simulink model "prob09"  (R2020b)
settings: Solver=VariableStepAuto  StartTime=0.0  StopTime=10.0  RelTol=1e-3
libraries: simulink x6, powerlib x5, sdolib x1
settings Model: Creator=stkaravind  LastModifiedBy=stkaravind

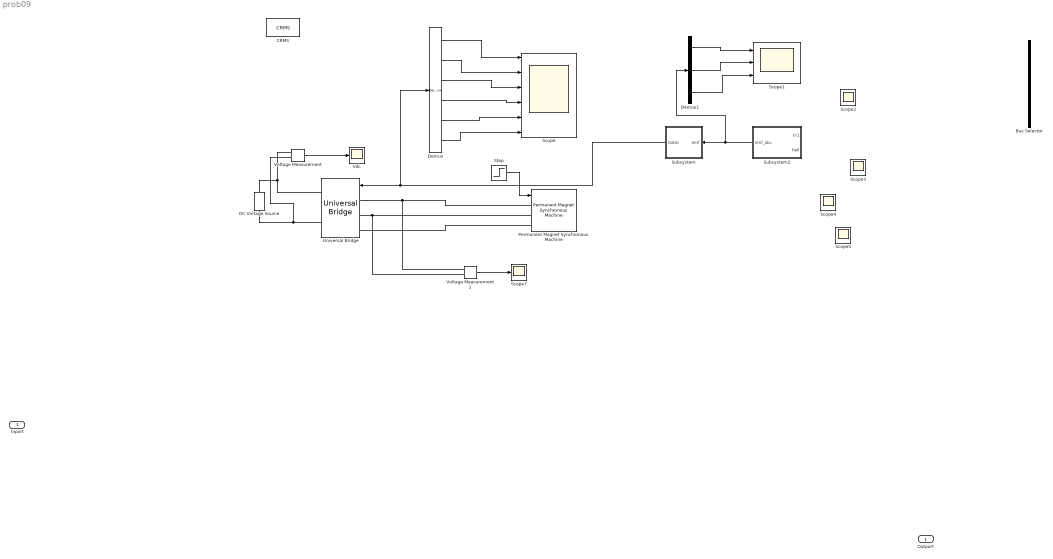
== system prob09 ==
  Inport : Inport
  Bus Selector : BusSelector  OutputSignals=signal1,signal2
  CRMS : sdolib/RMS Blocks/CRMS
      settings: SourceProductBaseCode=SO
  DC Voltage Source : powerlib/Electrical Sources/DC Voltage Source  Amplitude=300  Measurements=None
  Demux : Demux  Outputs=6
  Demux1 : Demux  Outputs=3
  Permanent Magnet Synchronous Machine : powerlib/Machines/Permanent Magnet Synchronous Machine  NbPhases=3  FluxDistribution=Trapezoidal  RotorType=Round  MechanicalLoad=Torque Tm  PresetModel=No  ShowDetailedParameters=on  MeasurementBus=off  Resistance=0.0485  Inductance=8.5e-3  dqInductances=[8.5e-3,8.5e-3]  La=0.000395  MachineConstant=Flux linkage established by magnets (V.s)  Flux=0.1194  VoltageCst=100.0283  TorqueCst=0.9552  Flat=120  Mechanical=[0.0027 0.0004924 4 0]  PolePairs=4  InitialConditions=[0,0, 0,0]  InitialConditions5ph=[0 0 0 0 0 0]  RefAngle=90 degrees behind phase A axis (modified Park)  IterativeDiscreteModel=Trapezoidal non iterative  TsBlock=-1  TsPowergui=0
  Scope : Scope  NumInputPorts=6
  Scope1 : Scope  NumInputPorts=3
  Scope{2..5,7} (5 alike) : Scope
  Step : Step  Time=.1  After=3  SampleTime=0
  Subsystem : Subsystem  TreatAsAtomicUnit=on
  Subsystem2 : Subsystem  TreatAsAtomicUnit=on
  Universal Bridge : powerlib/Power Electronics/Universal Bridge  Arms=3  SnubberResistance=5000  SnubberCapacitance=1e-6  Device=MOSFET / Diodes  Ron=1e-3  Lon=0  ForwardVoltages="[  0  0  ]"  ForwardVoltage=0  GTOparameters=[ 10e-6 , 20e-6 ]  IGBTparameters=[ 1e-6 , 2e-6 ]  Measurements=None  Measurements_2=None  converterType=Rectifier
  Vdc : Scope
  Voltage Measurement : powerlib/Measurements/Voltage Measurement  PhasorSimulation=off  OutputType=Complex  PSBequivalent=0
  Voltage Measurement1 : powerlib/Measurements/Voltage Measurement  PhasorSimulation=off  OutputType=Complex  PSBequivalent=0
  Outport : Outport
  wires:
  Step/1 -> Permanent Magnet Synchronous Machine/1
  Voltage Measurement/1 -> Vdc/1
  Voltage Measurement1/1 -> Scope7/1
  Demux/1 -> Scope/1
  Demux/2 -> Scope/2
  Demux/3 -> Scope/3
  Demux/4 -> Scope/4
  Demux/5 -> Scope/5
  Demux/6 -> Scope/6
  Subsystem/1(Gates) -> Demux/1, Universal Bridge/1
  Subsystem2/1(emf_abc) -> Demux1/1, Subsystem/1(emf)
  Demux1/1 -> Scope1/1
  Demux1/2 -> Scope1/2
  Demux1/3 -> Scope1/3
  connections:
  DC Voltage Source/RConn1 -- Universal Bridge/RConn1 -- Voltage Measurement/LConn1
  DC Voltage Source/LConn1 -- Voltage Measurement/LConn2 -- Universal Bridge/RConn2
  Universal Bridge/LConn1 -- Voltage Measurement1/LConn1 -- Permanent Magnet Synchronous Machine/LConn1
  Permanent Magnet Synchronous Machine/LConn2 -- Voltage Measurement1/LConn2 -- Universal Bridge/LConn2
  Permanent Magnet Synchronous Machine/LConn3 -- Universal Bridge/LConn3

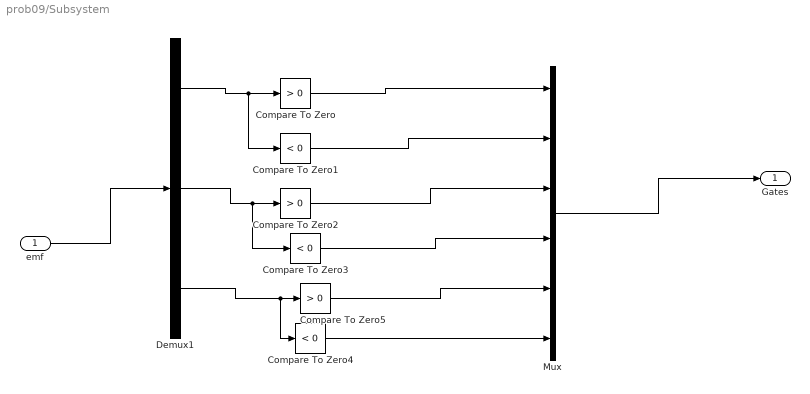
== system prob09/Subsystem ==
  emf : Inport
  Compare To Zero : simulink/Logic and Bit Operations/Compare To Zero  relop=>  OutDataTypeStr=boolean
  Compare To Zero1 : simulink/Logic and Bit Operations/Compare To Zero  relop=<  OutDataTypeStr=boolean
  Compare To Zero2 : simulink/Logic and Bit Operations/Compare To Zero  relop=>  OutDataTypeStr=boolean
  Compare To Zero3 : simulink/Logic and Bit Operations/Compare To Zero  relop=<  OutDataTypeStr=boolean
  Compare To Zero4 : simulink/Logic and Bit Operations/Compare To Zero  relop=<  OutDataTypeStr=boolean
  Compare To Zero5 : simulink/Logic and Bit Operations/Compare To Zero  relop=>  OutDataTypeStr=boolean
  Demux1 : Demux  Outputs=3
  Mux : Mux  Inputs=6
  Gates : Outport
  wires:
  Compare To Zero1/1 -> Mux/2
  Compare To Zero2/1 -> Mux/3
  Compare To Zero4/1 -> Mux/6
  Compare To Zero5/1 -> Mux/5
  Mux/1 -> Gates/1
  emf/1 -> Demux1/1
  Demux1/3 -> Compare To Zero4/1, Compare To Zero5/1
  Compare To Zero3/1 -> Mux/4
  Demux1/1 -> Compare To Zero1/1, Compare To Zero/1
  Compare To Zero/1 -> Mux/1
  Demux1/2 -> Compare To Zero3/1, Compare To Zero2/1

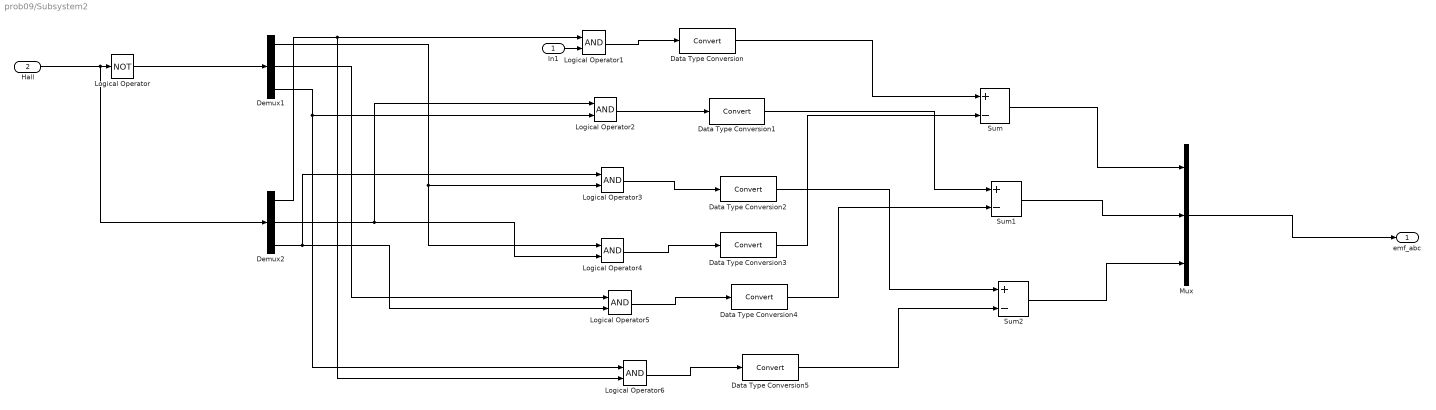
== system prob09/Subsystem2 ==
  In1 : Inport
  Hall : Inport  Port=2
  Data Type Conversion{,1..5} (6 alike) : DataTypeConversion
  Demux1 : Demux  Outputs=3
  Demux2 : Demux  Outputs=3
  Logical Operator : Logic  Operator=NOT  AllPortsSameDT=off  OutDataTypeStr=boolean
  Logical Operator{1..6} (6 alike) : Logic  AllPortsSameDT=off  OutDataTypeStr=boolean
  Mux : Mux  Inputs=3
  Sum : Sum  Inputs=+-
  Sum1 : Sum  Inputs=+-
  Sum2 : Sum  Inputs=+-
  emf_abc : Outport
  wires:
  Sum2/1 -> Mux/3
  Sum/1 -> Mux/1
  Data Type Conversion5/1 -> Sum2/2
  Logical Operator4/1 -> Data Type Conversion3/1
  Demux2/1 -> Logical Operator6/2, Logical Operator1/1
  Data Type Conversion2/1 -> Sum2/1
  Logical Operator5/1 -> Data Type Conversion4/1
  Mux/1 -> emf_abc/1
  Demux2/2 -> Logical Operator2/1, Logical Operator4/2
  Logical Operator1/1 -> Data Type Conversion/1
  Sum1/1 -> Mux/2
  Demux1/3 -> Logical Operator6/1, Logical Operator2/2
  Data Type Conversion4/1 -> Sum1/2
  Logical Operator3/1 -> Data Type Conversion2/1
  Demux1/2 -> Logical Operator5/1
  Data Type Conversion/1 -> Sum/1
  Hall/1 -> Demux2/1, Logical Operator/1
  Logical Operator2/1 -> Data Type Conversion1/1
  Demux1/1 -> Logical Operator4/1, Logical Operator3/2
  Logical Operator6/1 -> Data Type Conversion5/1
  Demux2/3 -> Logical Operator3/1, Logical Operator5/2
  Data Type Conversion3/1 -> Sum/2
  Data Type Conversion1/1 -> Sum1/1
  Logical Operator/1 -> Demux1/1
  In1/1 -> Logical Operator1/2
